simulink library "Electric_Drive_Simple_Efficiency"  (R2018b)
settings: Solver=VariableStepAuto  StartTime=0.0  StopTime=10.0  RelTol=1e-3
settings Model: Creator=Alexander Koch  LastModifiedBy=ga69qig
settings SFSimCC: SimUseLocalCustomCode=off
settings RTWCC: RTWUseLocalCustomCode=off
settings CodeAppCC: StateflowObjectComments=on

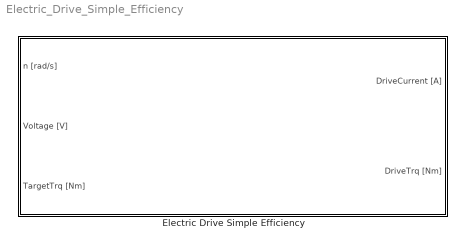
== system Electric_Drive_Simple_Efficiency ==
  Electric Drive Simple Efficiency : Subsystem  mask(SB){maxPower=100, maxRekuPower=-100, MaxTrq=60, Eff=0.97, LocalSampleTime=-1}
      mask prompts: maxPower "Maximal Mechanical Power [kW]"; maxRekuPower "Maximal Mechanical Rekuperation Power [kW]"; MaxTrq "Maximal Torque [Nm]"; Eff "Efficiency [-]"; LocalSampleTime "Local System Sample-Time [s]"
      mask help:
      | <Author> Alexander Koch, Benedikt Danquah based on Stefan Müller [1], Stephan Rohr [2]  </Author>
      |
      | <Date> 05/04/2017 </Date>
      |
      | <Description>
      | Voltage*Current*Efficiency = Rotation Speed * Drive Torque applies. The drive torque is limited by the maximal torque parameter and the maximal power. This means that higher rotational speeds can result in a lower driving torque.  Electrical power is higher by the factor 1/efficiency than the mechanical power in driving mode and lower in recuperation mode. Maximal recuperation power has to be negative
      | </Description>
      mask init:
      | GlobalSampleTime = CalcGlobalSampleTime(LocalSampleTime);
      mask Help:
      | <Parameters>
      | Maximal Mechanical Power [kW]
      | 	<Min> 0 </Min>
      | Maximal Rekuperation Power [kW]
      | 	<Max> 0 </Max>
      | Maximal Torque [Nm]
      | 	<Min> 0 </Min>
      | Efficiency [-]
      | 	<Max> 1 </Max>
      | 	<Min> 0 </Min>
      | Local System Sample-Time [s]
      | 	<Min> GlobalSampleTime </Min>
      | Global Sample-Time [s]
      | </Parameters>
      | 
      | <Inputs>
      | n [rad/s]
      | Voltage [V]
      | TargetTrq [Nm]
      | 	<sign orientation> [+] electric consumer </sign orientation>
      | </Inputs>
      | 
      | <Outputs>
      | DriveCurrent [A]
      | 	<sign orientation> [+] electric consumer </sign orientation>
      | DriveTrq [Nm]
      | </Outputs>
      | 
      | <Sources>
      | [1] S. Mueller, S. Rohr, W. Schmid, and M. Lienkamp, “Analysing the Influence of Driver Behaviour and Tuning Measures on Battery Aging and Residual Value of Electric Vehicles,” in Proc. EVS30 Symposium, Stuttgart, 2017, pp. 1–12.
      | [2] S. Rohr, “Technisch-wirtschaftliche Analyse des Zweitnutzungs- potentials von Lithium-Ionen-Traktionsbatterien,” Dissertation, Institute of Automotive Technology, Technical University Munich, Munich, 2018.
      | </Sources>
      mask TypeOptions maxPower: MaxPower/Value | Saturation/UpperLimit
      mask TypeOptions maxRekuPower: Saturation/LowerLimit | MaxRekuPower/Value
      mask TypeOptions MaxTrq: Saturation1/UpperLimit
      mask TypeOptions Eff: Efficency/Value
      mask TypeOptions LocalSampleTime: n [rad//s]/SampleTime | Voltage [V]/SampleTime | TargetTrq [Nm]/SampleTime
      mask DialogControl Container3 Prompt: Documentation:
      mask DialogControl Control2 Prompt: %<MaskHelp>
      mask DialogControl Container5 Prompt: Sample Time
      mask Display:
      | [picturexpos,pictureypos,picturewidth,pictureheight] = ...
      |     CalcBlockPicturePosition(gcb,1,0.01,0.0,100,100); % calculating picture position depending on Block size and minimum margin size
      | image('Electric_Drive_Simple_Efficiency.svg',[picturexpos pictureypos picturewidth pictureheight]); % plot picture to block

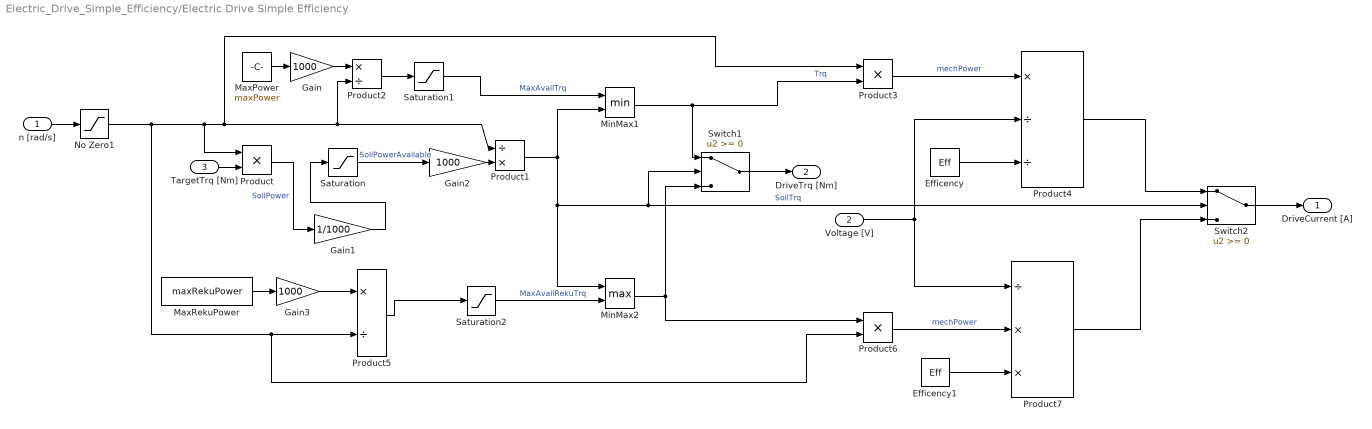
== system Electric_Drive_Simple_Efficiency/Electric Drive Simple Efficiency ==
  n [rad/s] : Inport  SampleTime=LocalSampleTime
  Voltage [V] : Inport  Port=2  SampleTime=LocalSampleTime
  TargetTrq [Nm] : Inport  Port=3  SampleTime=LocalSampleTime
  Efficency : Constant  Value=Eff
  Efficency1 : Constant  Value=Eff
  Gain : Gain  Gain=1000
  Gain1 : Gain  Gain=1/1000
  Gain2 : Gain  Gain=1000
  Gain3 : Gain  Gain=1000
  MaxPower : Constant  Value=maxPower
  MaxRekuPower : Constant  Value=maxRekuPower
  MinMax1 : MinMax  Inputs=2
  MinMax2 : MinMax  Function=max  Inputs=2
  No Zero1 : Saturate  UpperLimit=inf  LowerLimit=0.0001
  Product : Product
  Product1 : Product  Inputs=/*
  Product2 : Product  Inputs=*/
  Product3 : Product
  Product4 : Product  Inputs=*//
  Product5 : Product  Inputs=*/
  Product6 : Product
  Product7 : Product  Inputs=/**
  Saturation : Saturate  UpperLimit=maxPower  LowerLimit=maxRekuPower
  Saturation1 : Saturate  UpperLimit=MaxTrq  LowerLimit=0
  Saturation2 : Saturate  UpperLimit=0  LowerLimit=-MaxTrq
  Switch1 : Switch
  Switch2 : Switch
  DriveCurrent [A] : Outport  SampleTime=GlobalSampleTime
  DriveTrq [Nm] : Outport  Port=2  SampleTime=GlobalSampleTime
  wires:
  Product3/1 -> Product4/1  "mechPower"
  TargetTrq [Nm]/1 -> Product/2
  Product/1 -> Gain1/1  "SollPower"
  Voltage [V]/1 -> Product7/1, Product4/2
  Efficency/1 -> Product4/3
  Product1/1 -> Switch1/2, Switch2/2, MinMax2/1, MinMax1/2  "SollTrq"
  Product2/1 -> Saturation1/1
  Saturation1/1 -> MinMax1/1  "MaxAvailTrq"
  MinMax1/1 -> Switch1/1, Product3/2  "Trq"
  Saturation/1 -> Gain2/1  "SollPowerAvailable"
  MaxPower/1 -> Gain/1
  Product5/1 -> Saturation2/1
  n [rad/s]/1 -> No Zero1/1
  Saturation2/1 -> MinMax2/2  "MaxAvailRekuTrq"
  MaxRekuPower/1 -> Gain3/1
  MinMax2/1 -> Product6/1, Switch1/3
  Switch2/1 -> DriveCurrent [A]/1
  Product4/1 -> Switch2/1
  Switch1/1 -> DriveTrq [Nm]/1
  Product6/1 -> Product7/2  "mechPower"
  Efficency1/1 -> Product7/3
  No Zero1/1 -> Product1/1, Product2/2, Product3/1, Product/1, Product6/2, Product5/2
  Product7/1 -> Switch2/3
  Gain/1 -> Product2/1
  Gain1/1 -> Saturation/1
  Gain2/1 -> Product1/2
  Gain3/1 -> Product5/1
